simulink model "Design_5new_4weeks_Q3"  (R2026a)
settings: Solver=FixedStepAuto  StopTime=2419200  FixedStep=300
undefined symbols (not defined in the file): coloring, m, n, tamk, vapor
libraries: mqttlib x7
(part 2 of 2)

== matlab function Design_5new_4weeks_Q3/MATLAB Function2 ==
  data: d input; payload output double size=1


%function payload = fcn(d)
%#codegen

%payload = double(d);

%end

%%

%function payload = fcn(d)
%#codegen

%payload = 4.0;
%payload = uint8(4);
%payload = uint8('4');
%payload = uint8(52);   % '4'
%payload = '4';


%end


%%

function payload = fcn(d)
%#codegen

if d > 0
    payload = 4.0;   % Coloring completed
else
    payload = 0.0;
end

end

== matlab function Design_5new_4weeks_Q3/MATLAB Function3 ==
  data: d input; payload output double size=1

%function payload = fcn(d)


%function payload = fcn(d)
%#codegen

%if d > 0
  % payload = uint8(53);   % ASCII '5' = Vapor completed
%else
    %payload = uint8(48);   % ASCII '0' = no vapor yet
%end

%end

%%
%function payload = fcn(d)
%#codegen

%if d > 0
    %payload = 5.0;   % Vapor completed
%else
    %payload = 0.0;   % No vapor event
%end

%end

%%

function payload = fcn(d)
%#codegen

if d > 0
    payload = 5.0;   % Vapor completed
else
    payload = 0.0;
end

end
